simulink model "state2_manyUnitDelay"  (R2014a)
settings: Solver=FixedStepDiscrete  StartTime=0.0  StopTime=10.0  FixedStep=0.1  RelTol=1e-3
settings Model: Creator=yoshi12  LastModifiedBy=yoshi12

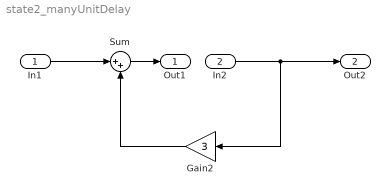
== system state2_manyUnitDelay ==
  In1 : Inport
  In2 : Inport  Port=2
  Gain2 : Gain  Gain=3
  Sum : Sum  Inputs=|++
  Out1 : Outport
  Out2 : Outport  Port=2
  wires:
  In2/1 -> Out2/1, Gain2/1
  Gain2/1 -> Sum/2
  In1/1 -> Sum/1
  Sum/1 -> Out1/1
